simulink model "LAB5"  (R2025b)
settings: Solver=VariableStepAuto  StartTime=0.0  StopTime=100  RelTol=1e-3
settings Model: Creator=Wingshingsho  LastModifiedBy=Wingshingsho

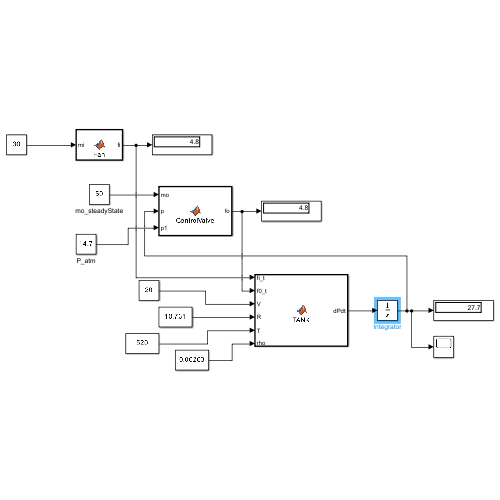
[thumbnail: Simulink's stored preview of the top-level diagram]
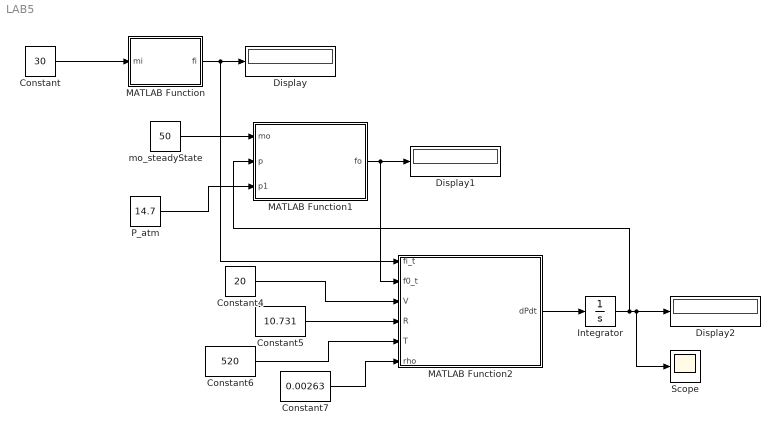
== system LAB5 ==
  Constant : Constant  Value=30
  Constant4 : Constant  Value=20
  Constant5 : Constant  Value=10.731
  Constant6 : Constant  Value=520
  Constant7 : Constant  Value=0.00263
  Display : Display
  Display1 : Display
  Display2 : Display
  Integrator : Integrator  InitialCondition=14.7
  MATLAB Function : MATLAB Function  TreatAsAtomicUnit=on
  MATLAB Function1 : MATLAB Function  TreatAsAtomicUnit=on
  MATLAB Function2 : MATLAB Function  TreatAsAtomicUnit=on
  P_atm : Constant  Value=14.7
  Scope : Scope
      settings: ActiveDisplayYMinimum=11.607550566516755  ActiveDisplayYMaximum=26.930880069191783
  mo_steadyState : Constant  Value=50
  wires:
  Constant/1 -> MATLAB Function/1(mi)
  MATLAB Function/1(fi) -> MATLAB Function2/1(fi_t), Display/1
  P_atm/1 -> MATLAB Function1/3(p1)
  MATLAB Function1/1(fo) -> MATLAB Function2/2(f0_t), Display1/1
  mo_steadyState/1 -> MATLAB Function1/1(mo)
  Constant4/1 -> MATLAB Function2/3(V)
  Constant5/1 -> MATLAB Function2/4(R)
  Constant6/1 -> MATLAB Function2/5(T)
  Constant7/1 -> MATLAB Function2/6(rho)
  MATLAB Function2/1(dPdt) -> Integrator/1
  Integrator/1 -> MATLAB Function1/2(p), Scope/1, Display2/1

== matlab function LAB5/MATLAB Function1 ==
  data: mo input; fo output; p input; p1 input
function fo = ControlValve(mo,p,p1)

fo = 0.00506 * mo * sqrt(p*(p-p1));

end

== matlab function LAB5/MATLAB Function ==
  data: mi input; fi output
function fi = Fan(mi)

fi = 0.16*mi;

end

== matlab function LAB5/MATLAB Function2 ==
  data: fi_t input; dPdt output; f0_t input; V input; R input; T input; rho input
function dPdt = TANK(fi_t,f0_t,V,R,T,rho)

dPdt = (R*T / V) * rho * (fi_t - f0_t);
end
